simulink model "forloop"  (R2021a)
settings: Solver=FixedStepDiscrete  StartTime=0.0  StopTime=10.0  RelTol=1e-3
settings Model: Creator=LEGION  LastModifiedBy=LEGION
settings OptimizationCC: DefaultParameterBehavior=Inlined  EnhancedBackFolding=on  PassReuseOutputArgsAs=Individual arguments  ZeroExternalMemoryAtStartup=off  ZeroInternalMemoryAtStartup=off  OptimizeBlockOrder=speed  DifferentSizesBufferReuse=on  OptimizationCustomize=off  EfficientTunableParamExpr=on
settings DebuggingCC: ParameterTunabilityLossMsg=error
settings SFSimCC: MATLABDynamicMemAlloc=off
settings RTWCC: SystemTargetFile=ert.tlc  GenCodeOnly=on  TemplateMakefile=ert_default_tmf  GenerateReport=on  IncludeHyperlinkInReport=on  LaunchReport=on  GenerateTraceInfo=on
settings CodeAppCC: ForceParamTrailComments=on  IgnoreCustomStorageClasses=off  OperatorAnnotations=on  SimulinkDataObjDesc=on  SFDataObjDesc=on  InsertBlockDesc=on
settings ERTTargetCC: TargetLangStandard=C99 (ISO)  GenerateSampleERTMain=on  InlinedParameterPlacement=NonHierarchical  ERTCustomFileTemplate=example_file_process.tlc  EnableUserReplacementTypes=on

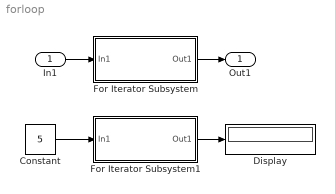
== system forloop ==
  In1 : Inport
  Constant : Constant  Value=5  OutDataTypeStr=uint16
  Display : Display
      settings: Format=decimal (Stored Integer)
  For Iterator Subsystem : Subsystem  TreatAsAtomicUnit=on
  For Iterator Subsystem1 : Subsystem  TreatAsAtomicUnit=on
  Out1 : Outport
  wires:
  In1/1 -> For Iterator Subsystem/1(In1)
  For Iterator Subsystem/1(Out1) -> Out1/1
  Constant/1 -> For Iterator Subsystem1/1(In1)
  For Iterator Subsystem1/1(Out1) -> Display/1

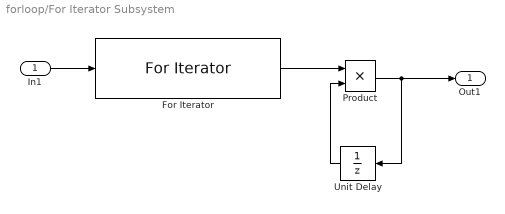
== system forloop/For Iterator Subsystem ==
  In1 : Inport  OutDataTypeStr=uint16
  For Iterator : ForIterator  IterationSource=external  IterationVariableDataType=uint16
  Product : Product  OutDataTypeStr=uint16
  Unit Delay : UnitDelay  InitialCondition=1  SampleTime=-1  HasFrameUpgradeWarning=on
  Out1 : Outport  OutDataTypeStr=uint16
  wires:
  In1/1 -> For Iterator/1
  Product/1 -> Unit Delay/1, Out1/1
  For Iterator/1 -> Product/1
  Unit Delay/1 -> Product/2

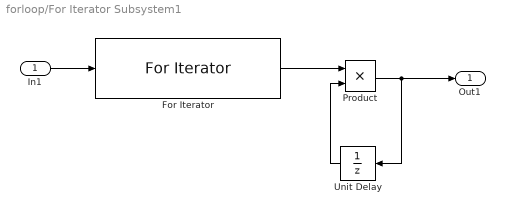
== system forloop/For Iterator Subsystem1 ==
  In1 : Inport  OutDataTypeStr=uint16
  For Iterator : ForIterator  IterationSource=external  IterationVariableDataType=uint16
  Product : Product  OutDataTypeStr=uint16
  Unit Delay : UnitDelay  InitialCondition=1  SampleTime=-1  HasFrameUpgradeWarning=on
  Out1 : Outport  OutDataTypeStr=uint16
  wires:
  In1/1 -> For Iterator/1
  Product/1 -> Unit Delay/1, Out1/1
  For Iterator/1 -> Product/1
  Unit Delay/1 -> Product/2
